simulink library "rateLimiter"  (R2016b)
settings: Solver=VariableStepAuto  StartTime=0.0  StopTime=10.0  RelTol=1e-3
undefined symbols (not defined in the file): CAL_fallingStep_pwmPerSample, CAL_risingStep_pwmPerSample
settings Model: Creator=oelkawok  LastModifiedBy=oelkawok

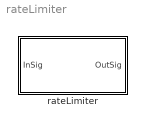
== system rateLimiter ==
  rateLimiter : Subsystem

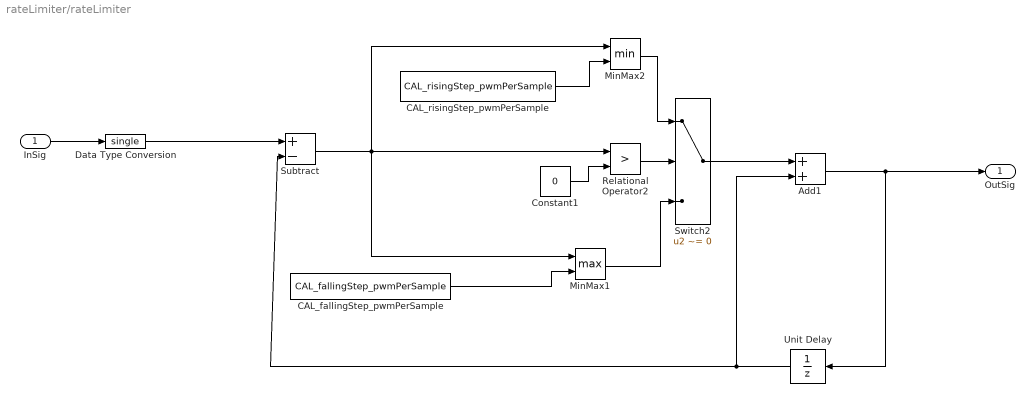
== system rateLimiter/rateLimiter ==
  InSig : Inport
  Add1 : Sum
  CAL_fallingStep_pwmPerSample : Constant  Value=CAL_fallingStep_pwmPerSample
  CAL_risingStep_pwmPerSample : Constant  Value=CAL_risingStep_pwmPerSample
  Constant1 : Constant  Value=0
  Data Type Conversion : DataTypeConversion  OutDataTypeStr=single
  MinMax1 : MinMax  Function=max  Inputs=2
  MinMax2 : MinMax  Inputs=2
  Relational Operator2 : RelationalOperator  Operator=>  OutDataTypeStr=boolean  RndMeth=Simplest
  Subtract : Sum  Inputs=+-
  Switch2 : Switch  Criteria=u2 ~= 0
  Unit Delay : UnitDelay  SampleTime=-1
  OutSig : Outport  OutputWhenDisabled=reset  InitialOutput=0
      settings: AttributesFormatString=|
      | Mode: %<OutputWhenDisabled>
      | init: %<InitialOutput>
  wires:
  Constant1/1 -> Relational Operator2/2
  Subtract/1 -> Relational Operator2/1, MinMax1/1, MinMax2/1
  MinMax2/1 -> Switch2/1
  Relational Operator2/1 -> Switch2/2
  MinMax1/1 -> Switch2/3
  InSig/1 -> Data Type Conversion/1
  CAL_risingStep_pwmPerSample/1 -> MinMax2/2
  Switch2/1 -> Add1/1
  Unit Delay/1 -> Subtract/2, Add1/2
  Data Type Conversion/1 -> Subtract/1
  Add1/1 -> Unit Delay/1, OutSig/1
  CAL_fallingStep_pwmPerSample/1 -> MinMax1/2
